simulink model "robot"  (R2017a)
settings: Solver=ode45  StartTime=0.0  StopTime=0.07  FixedStep=0.1  RelTol=1e-12  EnableMultiTasking=on
settings Model: Creator=amal029_old  LastModifiedBy=amal029
settings SolverCC: ZeroCrossAlgorithm=Adaptive  AutoInsertRateTranBlk=on
settings DataIOCC: LimitDataPoints=on
settings OptimizationCC: LifeSpan=inf
settings DebuggingCC: AllowSymbolicDim=off  SFUnexpectedBacktrackingDiag=warning  SFNoUnconditionalDefaultTransitionDiag=warning  SFExecutionAtInitializationDiag=none
settings GRTTargetCC: TargetLangStandard=C89/C90 (ANSI)
settings ConfigComp: CovMetricSettings=dw  CovHtmlReporting=on  CovSaveCumulativeToWorkspaceVar=on  CovSaveSingleToWorkspaceVar=on  CovShowResultsExplorer=off  CovExternalEMLEnable=off

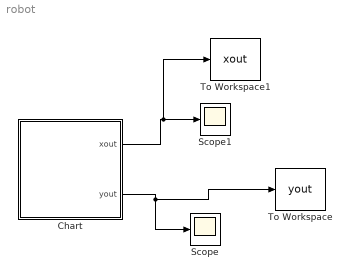
== system robot ==
  Chart : Stateflow chart  TreatAsAtomicUnit=on
  Scope : Scope
  Scope1 : Scope
  To Workspace : ToWorkspace  VariableName=yout  SampleTime=-1
      settings: Save2DSignal=2-D array (concatenate along first dimension)
  To Workspace1 : ToWorkspace  VariableName=xout  SampleTime=-1
      settings: Save2DSignal=2-D array (concatenate along first dimension)
  wires:
  Chart/2(yout) -> To Workspace/1, Scope/1
  Chart/1(xout) -> To Workspace1/1, Scope1/1

== stateflow chart robot/Chart ==
  settings: updateMethod=CONTINUOUS
  state State2
  state State1
    du:
    x_dot=cos(th)*30;
    y_dot=sin(th)*30;
    th_dot=tan(ph)/1*30;
    ph_dot=-10;
    xout=x;
    yout=y;
  State1 -> State2 : [(y>=1.8 && x<=2.8) || (y <= 0.8 && x <= 2.8)]
  (default) -> State1 : {x=0; y=1; th=0;ph=1; xout=x; yout=y;}
  data: x local; ph local; th local; y local; xout output; yout output
  data x settings: updateMethod=SF_CONTINUOUS_TIME_DATA
  data ph settings: updateMethod=SF_CONTINUOUS_TIME_DATA
  data th settings: updateMethod=SF_CONTINUOUS_TIME_DATA
  data y settings: updateMethod=SF_CONTINUOUS_TIME_DATA
